simulink model "pinpt_tester"  (Simulink 8.2)
settings: Solver=FixedStepDiscrete  SolverMode=SingleTasking  StartTime=0.0  StopTime=inf  FixedStep=0.0001  RelTol=1e-3
PostLoadFcn:
  | , if any(exist('dsrtsu_mdlpostloadfcn', 'file') == [2, 3, 6]), try dsrtsu_mdlpostloadfcn('Execute', bdroot); catch fprintf('Error in PostLoadFcn (dsrtsu_mdlpostloadfcn) for model "%s":\n %s\n', bdroot, lasterr); end, end,
libraries: ParsingLibrary x15, pinpt_decomposer_lib x1
settings Model: DSRTSU_INTERNAL_RTI_VER=440  DSRTSU_INTERNAL_RTI_TYPE=rti1401  DSRTSU_INTERNAL_RTIFPGA=30  Creator=Scott  LastModifiedBy=leidos  BufferReuse=off
settings OptimizationCC: BlockReduction=off  ConditionallyExecuteInputs=off  OptimizeBlockIOStorage=off  BufferReuse=off  ExpressionFolding=off  LocalBlockOutputs=off  InitFltsAndDblsToZero=on
settings DebuggingCC: FcnCallInpInsideContextMsg=EnableAllAsWarning  BusObjectLabelMismatch=none
settings HardwareCC: ProdIntDivRoundTo=Zero  ProdEndianess=BigEndian  ProdHWDeviceType=Generic->Custom  TargetIntDivRoundTo=Zero  TargetEndianess=BigEndian  TargetHWDeviceType=Generic->Custom
settings RTWCC: SystemTargetFile=rti1401.tlc  MakeCommand=make_rti  TemplateMakefile=rti1401.tmf  Description=dSPACE DS1401 Hardware Platform  ProcessScript=rti1401_make_rtw_hook  BuildConfiguration=Specify
settings STFCustomTargetCC: CodeReplacementLibrary=ANSI_C  ParMdlRefBuildCompliant=on  GeneratePreprocessorConditionals=Disable all  SystemTargetFile=rti1401.tlc
settings GRTTargetCC: CompOptLevelCompliant=off  ConcurrentExecutionCompliant=off  MatFileLogging=off  ExtModeMexFile=noextcomm
settings CustomProperty: DataType=RTWOptions_EnumType_C__Program Files_dSPACE RCPHIL 2014-A_MATLAB_RTI_RTI1401_TLC_rti1401_1InitialSimState  Value=RUN
settings EnumStrPairs: String=RUN

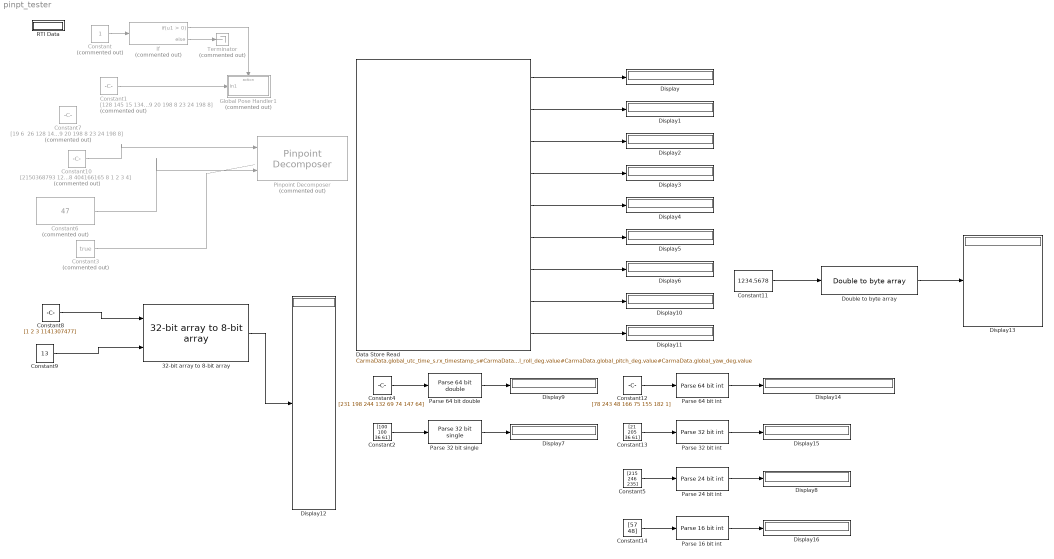
== system pinpt_tester ==
  32-bit array to 8-bit array : ParsingLibrary/32-bit array to 8-bit array
  Constant : Constant  Commented=on
  Constant1 : Constant  Commented=on  Value=[128 145 15 134 72 112 0 0 174 109 198 8 13 14 15 16 17 18 19 20 198 8 23 24 198 8]  OutDataTypeStr=uint8  SampleTime=0.05
  Constant10 : Constant  Commented=on  Value=[2150368793 1216745361 2919235696 218678893 218678893 353637138 404166165 8 1 2 3 4]  OutDataTypeStr=uint32  SampleTime=0.05
  Constant11 : Constant  Value=1234.5678  OutDataTypeStr=double  SampleTime=0.05
  Constant12 : Constant  Value=[78 243 48 166 75 155 182 1]  OutDataTypeStr=uint8  SampleTime=0.05
  Constant13 : Constant  Value=[21 205 36 61]  OutDataTypeStr=uint8  SampleTime=0.05
  Constant14 : Constant  Value=[57 48]  OutDataTypeStr=uint8  SampleTime=0.05
  Constant2 : Constant  Value=[100 100 36 61]  OutDataTypeStr=uint8  SampleTime=0.05
  Constant3 : Constant  Commented=on  Value=true
  Constant4 : Constant  Value=[231 198 244 132 69 74 147 64]  OutDataTypeStr=uint8  SampleTime=0.05
  Constant5 : Constant  Value=[215 246 235]  OutDataTypeStr=uint8  SampleTime=0.05
  Constant6 : Constant  Commented=on  Value=47  OutDataTypeStr=int32
  Constant7 : Constant  Commented=on  Value="[19 6  26 128 145 15 134 72 112 0 0 174 109 198 8 13 14 15 16 17 18 19 20 198 8 23 24 198 8]"  OutDataTypeStr=uint8  SampleTime=0.05
  Constant8 : Constant  Value=[1 2 3 1141307477]  OutDataTypeStr=uint32  SampleTime=0.05
  Constant9 : Constant  Value=13  SampleTime=0.05
  Data Store Read : DataStoreRead  DataStoreName=CarmaData  SampleTime=0.1  DataStoreElements=CarmaData.global_utc_time_s.rx_timestamp_s#CarmaData.global_utc_time_s.value#CarmaData.global_lat_deg.value#CarmaData.global_long_deg.value#CarmaData.global_alt_m.value#CarmaData.global_roll_deg.rx_timestamp_s#CarmaData.global_roll_deg.value#CarmaData.global_pitch_deg.value#CarmaData.global_yaw_deg.value
  Display{,1..16} (17 alike) : Display
      Display15 settings: Decimation=1.00
      Display16 settings: Decimation=1.00
      Display8 settings: Decimation=1.00
  "Double to byte array " : ParsingLibrary/Double to byte array 
  Global Pose Handler1 : Subsystem  Commented=on  TreatAsAtomicUnit=on
  If : If  Commented=on
  Parse 16 bit int : ParsingLibrary/Parse 16 bit int  Value=[0:1]  InDataTypeStr=uint16  factor=1  OutDataTypeStr=single
  Parse 24 bit int : ParsingLibrary/Parse 24 bit int  Value2=[0:2]  OutDataTypeStr=double  InDataTypeStr=int32  Value=1
  Parse 32 bit int : ParsingLibrary/Parse 32 bit int  Value2=[0:3]  OutDataTypeStr=double  InDataTypeStr=uint32  Value=1 / 1000
  Parse 32 bit single : ParsingLibrary/Parse 32 bit single  Value=[0:3]  Flip=False  factor=1  OutDataTypeStr=single
  Parse 64 bit double : ParsingLibrary/Parse 64 bit double  Value=[0:7]  factor=1  OutDataTypeStr=double
  Parse 64 bit int : ParsingLibrary/Parse 64 bit int  Value=[0:7]  factor=1/ 1000000  OutDataTypeStr=double
  Pinpoint Decomposer : pinpt_decomposer_lib/Pinpoint Decomposer  Commented=on
  RTI Data : Subsystem  Tag=struct('RTIDataServer',struct('RTIDataServerVs','2','RTIModelDescription','struct(''main'',''pinpt_tester'',''sub'','''',''isMp'',0)'))  LoadFcn="if exist('rtidc'), try,  rtidc('DataHostBlockClbLoad', gcbh); catch, disp(['Warning: ''LoadFcn'' for RTI Data block failed: ' lasterr]); end, end,"  mask(RTI_DATA_HOST){}
      mask help:
      | RTI Data Block.
      | This block is used by RTI to store internal model-dependent data.
      | Please keep this block on the root level of the model. Deleting this block will result in data loss.
      |
      | NEVER DELETE OR COPY THIS BLOCK!
      settings: CopyFcn="if exist('rtidc'), try,  rtidc('DataHostBlockClbCopy', gcbh); catch, disp(['Warning: ''CopyFcn'' for RTI Data block failed: ' lasterr]); end, end,"  DeleteFcn="if exist('rtidc'), try,  rtidc('DataHostBlockClbDelete', gcbh); catch, disp(['Warning: ''DeleteFcn'' for RTI Data block failed: ' lasterr]); end, end,"  ModelCloseFcn="if exist('rtidc'), try,  rtidc('DataHostBlockClbModelClose', gcbh); catch, disp(['Warning: ''ModelCloseFcn'' for RTI Data block failed: ' lasterr]); end, end,"  PreSaveFcn="if exist('rtidc'), try,  rtidc('DataHostBlockClbPreSave', gcbh); catch, disp(['Warning: ''PreSaveFcn'' for RTI Data block failed: ' lasterr]); end, end,"  PostSaveFcn="if exist('rtidc'), try,  rtidc('DataHostBlockClbPostSave', gcbh); catch, disp(['Warning: ''PostSaveFcn'' for RTI Data block failed: ' lasterr]); end, end,"  NameChangeFcn="if exist('rtidc'), try,  rtidc('DataHostBlockClbNameChange', gcbh); catch, disp(['Warning: ''NameChangeFcn'' for RTI Data block failed: ' lasterr]); end, end,"
      mask Help:
      | RTI Data Block.
      | This block is used by RTI to store internal model-dependent data.
      | Please keep this block on the root level of the model. Deleting this block will result in data loss.
      | 
      | NEVER DELETE OR COPY THIS BLOCK!
      mask Display:
      | text(0.5, 0.5, 'RTI Data', 'HorizontalAlignment', 'center');
      | plot([1 0]);
  Terminator : Terminator  Commented=on
  wires:
  If/2 -> Terminator/1
  Constant/1 -> If/1
  If/1 -> Global Pose Handler1/Action
  Constant1/1 -> Global Pose Handler1/1(In1)
  Data Store Read/1 -> Display/1
  Data Store Read/2 -> Display1/1
  Data Store Read/3 -> Display2/1
  Data Store Read/4 -> Display3/1
  Data Store Read/5 -> Display4/1
  Data Store Read/6 -> Display5/1
  Data Store Read/7 -> Display6/1
  Parse 32 bit single/1 -> Display7/1
  Constant2/1 -> Parse 32 bit single/1
  Parse 24 bit int/1 -> Display8/1
  Constant5/1 -> Parse 24 bit int/1
  Constant4/1 -> Parse 64 bit double/1
  Parse 64 bit double/1 -> Display9/1
  Data Store Read/8 -> Display10/1
  Data Store Read/9 -> Display11/1
  Constant3/1 -> ?
  Constant10/1 -> Pinpoint Decomposer/1
  Constant6/1 -> Pinpoint Decomposer/2
  Constant8/1 -> 32-bit array to 8-bit array/1
  Constant9/1 -> 32-bit array to 8-bit array/2
  32-bit array to 8-bit array/1 -> Display12/1
  Constant11/1 -> "Double to byte array "/1
  "Double to byte array "/1 -> Display13/1
  Constant12/1 -> Parse 64 bit int/1
  Parse 64 bit int/1 -> Display14/1
  Parse 32 bit int/1 -> Display15/1
  Constant13/1 -> Parse 32 bit int/1
  Parse 16 bit int/1 -> Display16/1
  Constant14/1 -> Parse 16 bit int/1

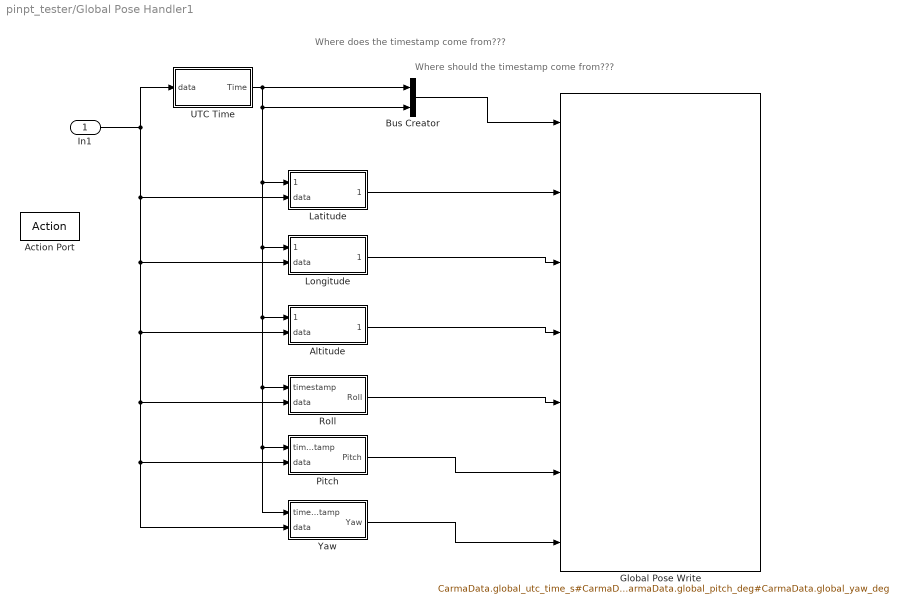
== system pinpt_tester/Global Pose Handler1 ==
  note: Where should the timestamp come from???
  note: Where does the timestamp come from???
  In1 : Inport
  Action Port : ActionPort  ActionType=then
  Altitude : Subsystem
  Bus Creator : BusCreator  Inputs=2  OutDataTypeStr=Bus: TimestampedDouble  NonVirtualBus=on
  Global Pose Write : DataStoreWrite  DataStoreName=CarmaData  DataStoreElements=CarmaData.global_utc_time_s#CarmaData.global_lat_deg#CarmaData.global_long_deg#CarmaData.global_alt_m#CarmaData.global_roll_deg#CarmaData.global_pitch_deg#CarmaData.global_yaw_deg
  Latitude : Subsystem
  Longitude : Subsystem
  Pitch : Subsystem
  Roll : Subsystem
  UTC Time : Subsystem
  Yaw : Subsystem
  wires:
  In1/1 -> Latitude/2(data), Longitude/2(data), Altitude/2(data), Roll/2(data), Pitch/2(data), Yaw/2(data), UTC Time/1(data)
  Latitude/1(Latitiude) -> Global Pose Write/2
  Longitude/1(Longitude) -> Global Pose Write/3
  Altitude/1(Altitude) -> Global Pose Write/4
  Roll/1(Roll) -> Global Pose Write/5
  Pitch/1(Pitch) -> Global Pose Write/6
  Yaw/1(Yaw) -> Global Pose Write/7
  UTC Time/1(Time) -> Yaw/1(timestamp), Pitch/1(timestamp), Roll/1(timestamp), Altitude/1(timestamp), Longitude/1(timestamp), Latitude/1(timestamp), Bus Creator/2, Bus Creator/1
  Bus Creator/1 -> Global Pose Write/1

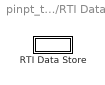
== system pinpt_tester/RTI Data ==
  RTI Data Store : Subsystem  Tag="struct('private',struct('version',struct('dsVer',uint32(2)),'access',struct('modified',['17-Aug-2015 19:03:02'],'type','Model','isPerm',1)),'public',struct('main',struct('data',[]),'sub',struct('name',{{'pinpt_tester'}},'data',{{struct('TH',struct('thTaskInfo',struct('taskType',{'TIMER','HWINT','TMRINT','SWINT','GLINT'},'tasksNumOf',{1,0,0,0,0},'srcIds',{{'TIMERA'},{},{},{},{}},'taskNames',{{['Timer Task 1']},{},{},{},{}})),'th_tc',struct('dataType','TASK','taskGroupId','','taskGroupList',{{}},'taskSchedulingPolicy','FCFS','taskType','TIMER','blkh',-1,'srcId','TIMERA','srcSgnName',['Timer A interrupt'],'srcCpuName','','taskName',['Timer Task 1  [0.0001] s'],'taskNameDisplayExt','','smplTime',0.0001,'smplTimeOffs',0,'hasFixedPriority',0,'priority',1,'hasFixedOvc',0,'ovcType',1,'ovcMax',1),'tc_th',struct('dataType','TASK','taskGroupId','','taskGroupList',{{}},'taskSchedulingPolicy','FCFS','taskType','TIMER','blkh',-1,'srcId','TIMERA','srcSgnName',['Timer A interrupt'],'srcCpuName','','taskName',['Timer Task 1  [0.0001] s'],'taskNameDisplayExt','','smplTime',0.0001,'smplTimeOffs',0,'hasFixedPriority',0,'priority',1,'hasFixedOvc',0,'ovcType',1,'ovcMax',1))}})))"  mask(RTI_DATA_STORE){}
      mask help:
      | RTI Data Store Block. This block is used by RTI to store internal model dependent data. Deleting this block will result in data loss.
      |
      | NEVER DELETE, COPY, OR MODIFY THIS BLOCK!
      mask Help:
      | RTI Data Store Block. This block is used by RTI to store internal model dependent data. Deleting this block will result in data loss.
      | 
      | NEVER DELETE, COPY, OR MODIFY THIS BLOCK!
      mask Display: text(0.5, 0.5, ' ', 'HorizontalAlignment', 'center');

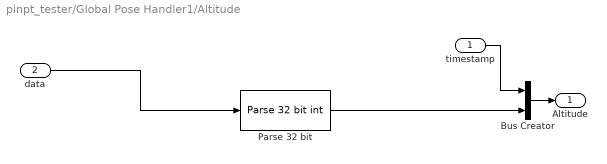
== system pinpt_tester/Global Pose Handler1/Altitude ==
  timestamp : Inport
  data : Inport  Port=2
  Bus Creator : BusCreator  Inputs=2  OutDataTypeStr=Bus: TimestampedDouble  NonVirtualBus=on
  Parse 32 bit : ParsingLibrary/Parse 32 bit int  Value2=[0:3]  OutDataTypeStr=double  InDataTypeStr=int32  Value=1/1000
  Altitude : Outport
  wires:
  Bus Creator/1 -> Altitude/1
  timestamp/1 -> Bus Creator/1
  data/1 -> Parse 32 bit/1
  Parse 32 bit/1 -> Bus Creator/2

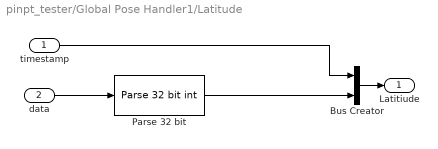
== system pinpt_tester/Global Pose Handler1/Latitude ==
  timestamp : Inport
  data : Inport  Port=2
  Bus Creator : BusCreator  Inputs=2  OutDataTypeStr=Bus: TimestampedDouble  NonVirtualBus=on
  Parse 32 bit : ParsingLibrary/Parse 32 bit int  Value2=[0:3]  OutDataTypeStr=double  InDataTypeStr=int32  Value=180.0 / 2^31
  Latitiude : Outport
  wires:
  Bus Creator/1 -> Latitiude/1
  timestamp/1 -> Bus Creator/1
  Parse 32 bit/1 -> Bus Creator/2
  data/1 -> Parse 32 bit/1

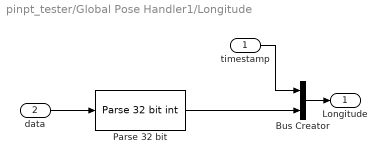
== system pinpt_tester/Global Pose Handler1/Longitude ==
  timestamp : Inport
  data : Inport  Port=2
  Bus Creator : BusCreator  Inputs=2  OutDataTypeStr=Bus: TimestampedDouble  NonVirtualBus=on
  Parse 32 bit : ParsingLibrary/Parse 32 bit int  Value2=[0:3]  OutDataTypeStr=double  InDataTypeStr=int32  Value=180.0 / 2^31
  Longitude : Outport
  wires:
  Bus Creator/1 -> Longitude/1
  timestamp/1 -> Bus Creator/1
  Parse 32 bit/1 -> Bus Creator/2
  data/1 -> Parse 32 bit/1

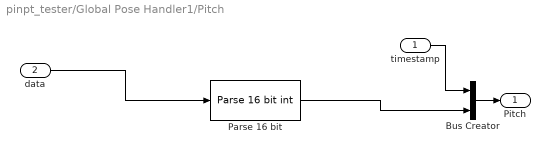
== system pinpt_tester/Global Pose Handler1/Pitch ==
  timestamp : Inport
  data : Inport  Port=2
  Bus Creator : BusCreator  Inputs=2  OutDataTypeStr=Bus: TimestampedSingle  NonVirtualBus=on
  Parse 16 bit : ParsingLibrary/Parse 16 bit int  Value=180 / 2^15  InDataTypeStr=int16  factor=1  OutDataTypeStr=single
  Pitch : Outport
  wires:
  Bus Creator/1 -> Pitch/1
  timestamp/1 -> Bus Creator/1
  data/1 -> Parse 16 bit/1
  Parse 16 bit/1 -> Bus Creator/2

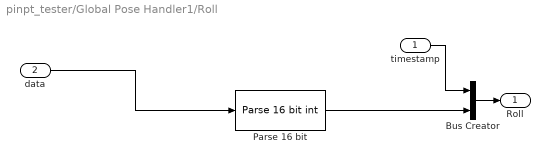
== system pinpt_tester/Global Pose Handler1/Roll ==
  timestamp : Inport
  data : Inport  Port=2
  Bus Creator : BusCreator  Inputs=2  OutDataTypeStr=Bus: TimestampedSingle  NonVirtualBus=on
  Parse 16 bit : ParsingLibrary/Parse 16 bit int  Value=180 / 2^15  InDataTypeStr=int16  factor=1  OutDataTypeStr=single
  Roll : Outport
  wires:
  Bus Creator/1 -> Roll/1
  timestamp/1 -> Bus Creator/1
  data/1 -> Parse 16 bit/1
  Parse 16 bit/1 -> Bus Creator/2

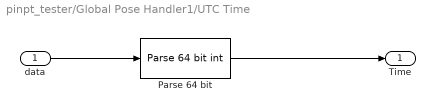
== system pinpt_tester/Global Pose Handler1/UTC Time ==
  data : Inport
  Parse 64 bit : ParsingLibrary/Parse 64 bit int  Value=1 / 1000000  factor=1  OutDataTypeStr=double
  Time : Outport
  wires:
  data/1 -> Parse 64 bit/1
  Parse 64 bit/1 -> Time/1

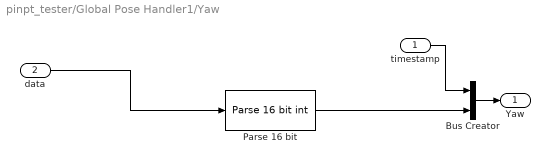
== system pinpt_tester/Global Pose Handler1/Yaw ==
  timestamp : Inport
  data : Inport  Port=2
  Bus Creator : BusCreator  Inputs=2  OutDataTypeStr=Bus: TimestampedSingle  NonVirtualBus=on
  Parse 16 bit : ParsingLibrary/Parse 16 bit int  Value=180 / 2^15  InDataTypeStr=int16  factor=1  OutDataTypeStr=single
  Yaw : Outport
  wires:
  Bus Creator/1 -> Yaw/1
  timestamp/1 -> Bus Creator/1
  data/1 -> Parse 16 bit/1
  Parse 16 bit/1 -> Bus Creator/2

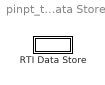
== system pinpt_tester/RTI Data/RTI Data Store ==
  RTI Data Store : Subsystem  mask(RTI_DATA_STORE){}
      mask help:
      | RTI Data Store Block. This block is used by RTI to store internal model dependent data. Deleting this block will result in data loss.
      |
      | NEVER DELETE, COPY, OR MODIFY THIS BLOCK!
      mask Help:
      | RTI Data Store Block. This block is used by RTI to store internal model dependent data. Deleting this block will result in data loss.
      | 
      | NEVER DELETE, COPY, OR MODIFY THIS BLOCK!
      mask Display: text(0.5, 0.5, ' ', 'HorizontalAlignment', 'center');

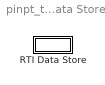
== system pinpt_tester/RTI Data/RTI Data Store/RTI Data Store ==
  RTI Data Store : Subsystem  mask(RTI_DATA_STORE){}
      mask help:
      | RTI Data Store Block. This block is used by RTI to store internal model dependent data. Deleting this block will result in data loss.
      |
      | NEVER DELETE, COPY, OR MODIFY THIS BLOCK!
      mask Help:
      | RTI Data Store Block. This block is used by RTI to store internal model dependent data. Deleting this block will result in data loss.
      | 
      | NEVER DELETE, COPY, OR MODIFY THIS BLOCK!
      mask Display: text(0.5, 0.5, ' ', 'HorizontalAlignment', 'center');

== system pinpt_tester/RTI Data/RTI Data Store/RTI Data Store/RTI Data Store ==
  RTI Data Store : Subsystem  mask(RTI_DATA_STORE){}
      mask help:
      | RTI Data Store Block. This block is used by RTI to store internal model dependent data. Deleting this block will result in data loss.
      |
      | NEVER DELETE, COPY, OR MODIFY THIS BLOCK!
      mask Help:
      | RTI Data Store Block. This block is used by RTI to store internal model dependent data. Deleting this block will result in data loss.
      | 
      | NEVER DELETE, COPY, OR MODIFY THIS BLOCK!
      mask Display: text(0.5, 0.5, ' ', 'HorizontalAlignment', 'center');

== system pinpt_tester/RTI Data/RTI Data Store/RTI Data Store/RTI Data Store/RTI Data Store ==
